simulink model "vexarmcortex_BEST_IR_Sensor_Counter"  (R2019a)
settings: Solver=FixedStepAuto  StartTime=0.0  StopTime=inf  RelTol=1e-3  EnableMultiTasking=on
libraries: simulink x1, vexarmcortexlib x1
settings Model: SimulationMode=external  ExtModeTrigDuration=25  Creator=The MathWorks, Inc.  LastModifiedBy=josea
settings DataIOCC: ReturnWorkspaceOutputs=off
settings OptimizationCC: MaxStackSize=64
settings DebuggingCC: ParameterTunabilityLossMsg=error  ArithmeticOperatorsInVariantConditions=warning
settings HardwareCC: ProdBitPerPointer=32  ProdBitPerSizeT=32  ProdBitPerPtrDiffT=32  ProdLargestAtomicInteger=Long  ProdLargestAtomicFloat=Double  ProdWordSize=32  ProdHWDeviceType=ARM Compatible->ARM Cortex  UseEmbeddedCoderFeatures=off
settings SFSimCC: SimUseLocalCustomCode=off
settings RTWCC: SystemTargetFile=ert.tlc  HardwareBoard=ARM Cortex-based VEX Microcontroller  TLCOptions="-aInlineSetEventsForThisBaseRateFcn=TLC_FALSE -aSuppressMultiTaskScheduler=TLC_FALSE  -aRateBasedStepFcn=0"  TemplateMakefile=ert_default_tmf  RTWUseLocalCustomCode=off  Toolchain=GNU Tools for VEX ARM Cortex
settings CodeAppCC: ForceParamTrailComments=on  OperatorAnnotations=on  StateflowObjectComments=on  MATLABSourceComments=on
settings ERTTargetCC: ERTCustomFileBanners=off  SupportContinuousTime=on  SupportNonInlinedSFcns=on  RemoveResetFunc=off  ModelStepFunctionPrototypeControlCompliant=off

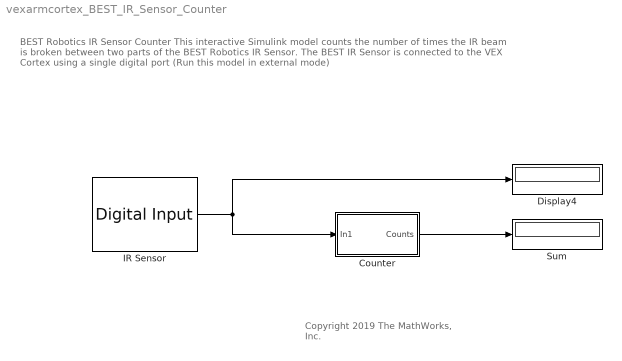
== system vexarmcortex_BEST_IR_Sensor_Counter ==
  note: BEST Robotics IR Sensor Counter
      | This interactive Simulink model counts the number of times the IR beam is broken between
      | two parts of the BEST Robotics IR Sensor. The BEST IR Sensor is connected to the VEX Cortex
      | using a single digital port (Run this model in external mode)
  note: Copyright 2019 The MathWorks, Inc.
  Counter : Subsystem
  Display4 : Display
  IR Sensor : vexarmcortexlib/Sensors/Digital Input  inChan=1  SimulationIn=off  SampleTime=0.05
      settings: SourceProductName=Simulink Coder Support Package for ARM Cortex-based VEX Microcontroller  SourceProductBaseCode=EC_VEX_MICRO
  Sum : Display
  wires:
  IR Sensor/1 -> Counter/1(In1), Display4/1
  Counter/1(Counts) -> Sum/1

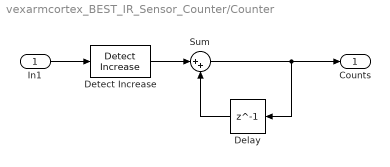
== system vexarmcortex_BEST_IR_Sensor_Counter/Counter ==
  In1 : Inport
  Delay : Delay  DelayLength=1
  Detect Increase : simulink/Logic and Bit Operations/Detect Increase  vinit=0.0  OutDataTypeStr=uint8
  Sum : Sum  Inputs=|++
  Counts : Outport
  wires:
  In1/1 -> Detect Increase/1
  Detect Increase/1 -> Sum/1
  Sum/1 -> Delay/1, Counts/1
  Delay/1 -> Sum/2
